simulink model "Movimiento_rotacional_simulink_1"  (R2022b)
settings: Solver=VariableStepAuto  StartTime=0.0  StopTime=10.0  MaxStep=.0001  RelTol=1e-3
values from neighbouring files (symbols this model uses):
  k = 100    [DobleP3_1.m]
  m = 10    [DobleP3_1.m]
  r = 0.05    [DobleP3_1.m]
settings Model: Creator=bryan  LastModifiedBy=mluser

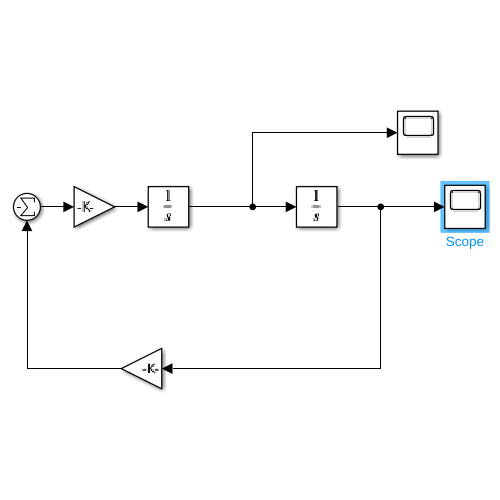
[thumbnail: Simulink's stored preview of the top-level diagram]
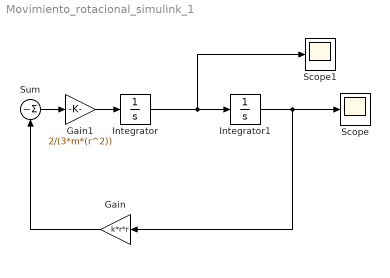
== system Movimiento_rotacional_simulink_1 ==
  Gain : Gain  Gain=k*r*r
  Gain1 : Gain  Gain=2/(3*m*(r^2))
  Integrator : Integrator  InitialCondition=2
  Integrator1 : Integrator
  Scope : Scope
  Scope1 : Scope
  Sum : Sum  Inputs=|-
  wires:
  Integrator/1 -> Scope1/1, Integrator1/1
  Integrator1/1 -> Gain/1, Scope/1
  Sum/1 -> Gain1/1
  Gain/1 -> Sum/1
  Gain1/1 -> Integrator/1
